simulink model "SendSimpleTest"  (R2015b)
settings: Solver=VariableStepAuto  StartTime=0.0  StopTime=inf  RelTol=1e-3
libraries: simulink x1, dspnetwork x1, aerolibanimutils x1
settings Model: Creator=Ryuu  LastModifiedBy=Ryuu

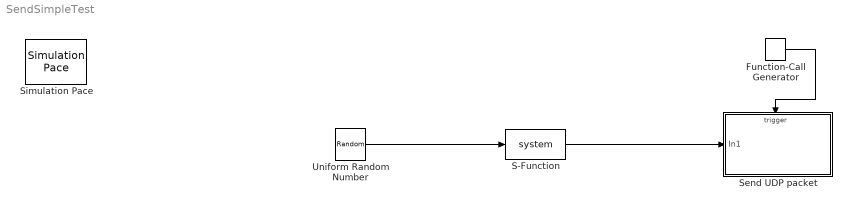
== system SendSimpleTest ==
  Function-Call Generator : simulink/Ports & Subsystems/Function-Call Generator  sample_time=.5  numberOfIterations=1
  S-Function : S-Function  SFunctionDeploymentMode=off  EnableBusSupport=off
  Send UDP packet : Subsystem
  Simulation Pace : aerolibanimutils/Simulation Pace  SimulationPace=1  SleepMode=MATLAB Thread  OutputPaceError=off  SampleTime=1/30
  Uniform Random Number : UniformRandomNumber  Maximum=100  SampleTime=0.1
  wires:
  Function-Call Generator/1 -> Send UDP packet/Trigger
  Uniform Random Number/1 -> S-Function/1
  S-Function/1 -> Send UDP packet/1(In1)

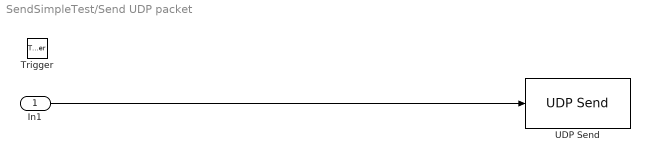
== system SendSimpleTest/Send UDP packet ==
  In1 : Inport
  Trigger : TriggerPort  TriggerType=function-call  PortDimensions=1
  UDP Send : dspnetwork/UDP Send  remoteURL='127.0.0.1'  remotePort=25000  localURL='0.0.0.0'  localPortSource=Automatically determine  localPort=-1  sampletime=-1  separateLengthPort=0
  wires:
  In1/1 -> UDP Send/1
